simulink model "motor_model"  (R2022b)
settings: Solver=VariableStepAuto  StartTime=0.0  StopTime=5  FixedStep=Ts  RelTol=1e-3
undefined symbols (not defined in the file): DiscIntNeverNeededParam, param
settings Model: Creator=adelk  LastModifiedBy=adelk

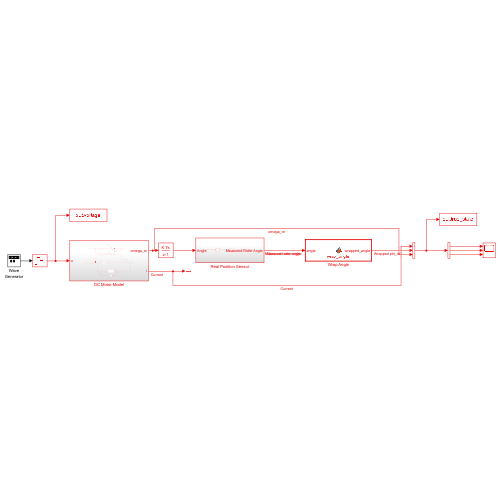
[thumbnail: Simulink's stored preview of the top-level diagram]
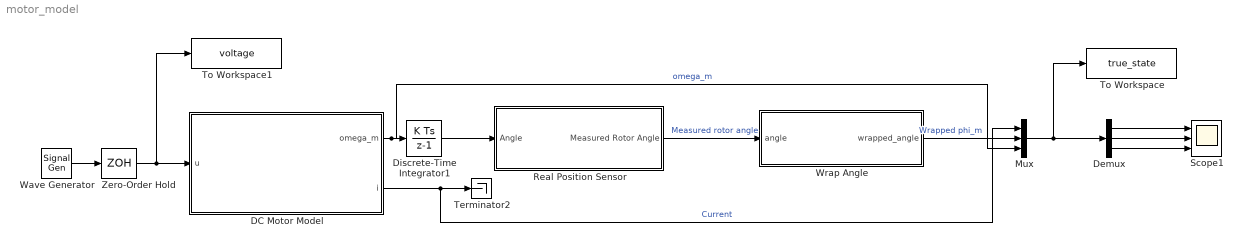
== system motor_model ==
  DC Motor Model : Subsystem
  Demux : Demux  Outputs=3
  Discrete-Time Integrator1 : DiscreteIntegrator  SampleTime=param.Ts  ICPrevOutput=DiscIntNeverNeededParam  ICPrevScaledInput=DiscIntNeverNeededParam
  Mux : Mux  Inputs=3
  Real Position Sensor : Subsystem
  Scope1 : Scope  NumInputPorts=3
  Terminator2 : Terminator
  To Workspace : ToWorkspace  VariableName=true_state  SampleTime=param.Ts
      settings: Save2DSignal=2-D array (concatenate along first dimension)
  To Workspace1 : ToWorkspace  VariableName=voltage  SampleTime=param.Ts
      settings: Save2DSignal=2-D array (concatenate along first dimension)
  Wave Generator : SignalGenerator  WaveForm=square  Amplitude=24  Frequency=50  Units=rad/sec
  Wrap Angle : MATLAB Function  TreatAsAtomicUnit=on
  Zero-Order Hold : ZeroOrderHold  SampleTime=param.Ts
  wires:
  DC Motor Model/1(omega_m) -> Mux/3, Discrete-Time Integrator1/1  "omega_m"
  DC Motor Model/2(i) -> Mux/1, Terminator2/1  "Current"
  Discrete-Time Integrator1/1 -> Real Position Sensor/1(Angle)
  Zero-Order Hold/1 -> To Workspace1/1, DC Motor Model/1(u)
  Real Position Sensor/1(Measured Rotor Angle) -> Wrap Angle/1(angle)  "Measured rotor angle"
  Mux/1 -> Demux/1, To Workspace/1
  Demux/1 -> Scope1/1
  Demux/2 -> Scope1/2
  Demux/3 -> Scope1/3
  Wrap Angle/1(wrapped_angle) -> Mux/2  "Wrapped phi_m"
  Wave Generator/1 -> Zero-Order Hold/1

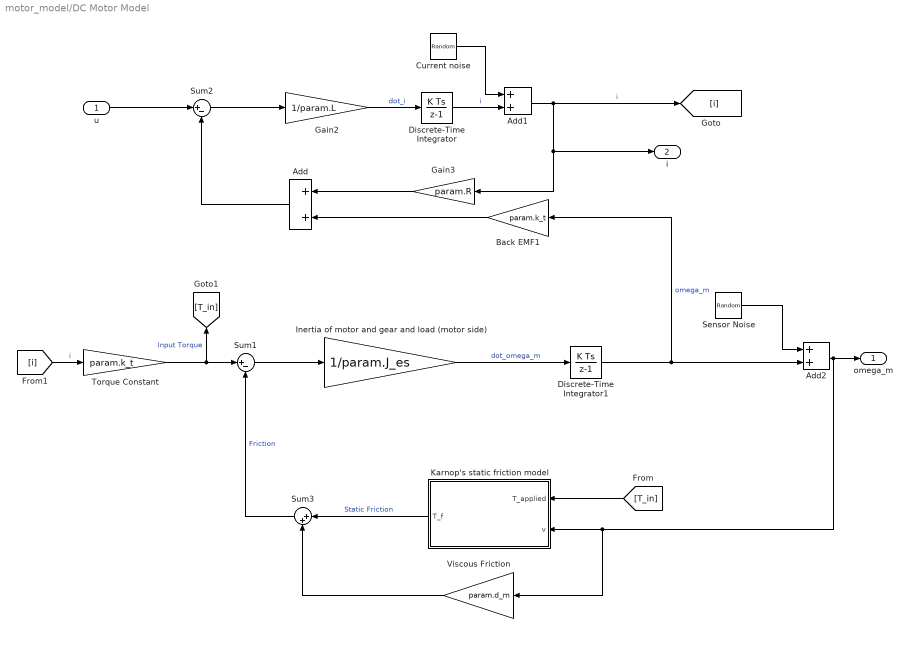
== system motor_model/DC Motor Model ==
  u : Inport
  Add : Sum
  Add1 : Sum
  Add2 : Sum
  Back EMF1 : Gain  Gain=param.k_t
  Current noise : RandomNumber  Variance=param.std_current_noise  SampleTime=param.Ts
  Discrete-Time Integrator : DiscreteIntegrator  SampleTime=param.Ts  ICPrevOutput=DiscIntNeverNeededParam  ICPrevScaledInput=DiscIntNeverNeededParam
  Discrete-Time Integrator1 : DiscreteIntegrator  SampleTime=param.Ts  ICPrevOutput=DiscIntNeverNeededParam  ICPrevScaledInput=DiscIntNeverNeededParam
  Gain2 : Gain  Gain=1/param.L
  Gain3 : Gain  Gain=param.R
  Inertia of motor and gear and load (motor side) : Gain  Gain=1/param.J_es
  Karnop's static friction model : Subsystem
  Sensor Noise : RandomNumber  Variance=param.std_encoder_noise  SampleTime=param.Ts
  Sum1 : Sum  Inputs=|+-
  Sum2 : Sum  Inputs=|+-
  Sum3 : Sum  Inputs=|++
  Torque Constant : Gain  Gain=param.k_t
  Viscous Friction : Gain  Gain=param.d_m
  omega_m : Outport
  i : Outport  Port=2
  wires:
  Add/1 -> Sum2/2
  Back EMF1/1 -> Add/2
  Gain3/1 -> Add/1
  Sum2/1 -> Gain2/1
  Add1/1 -> [i], Gain3/1, i/1  "i"
  Gain2/1 -> Discrete-Time Integrator/1  "dot_i"
  Inertia of motor and gear and load (motor side)/1 -> Discrete-Time Integrator1/1  "dot_omega_m"
  Discrete-Time Integrator1/1 -> Add2/2, Back EMF1/1  "omega_m"
  Torque Constant/1 -> [T_in], Sum1/1  "Input Torque"
  Viscous Friction/1 -> Sum3/2
  Sum1/1 -> Inertia of motor and gear and load (motor side)/1
  [i] -> Torque Constant/1  "i"
  Karnop's static friction model/1(T_f) -> Sum3/1  "Static Friction"
  Sum3/1 -> Sum1/2  "Friction"
  [T_in] -> Karnop's static friction model/1(T_applied)
  u/1 -> Sum2/1
  Discrete-Time Integrator/1 -> Add1/2  "i"
  Current noise/1 -> Add1/1
  Sensor Noise/1 -> Add2/1
  Add2/1 -> Viscous Friction/1, Karnop's static friction model/2(v), omega_m/1

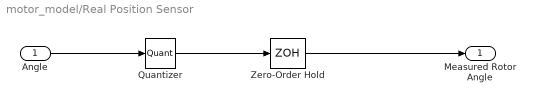
== system motor_model/Real Position Sensor ==
  Angle : Inport
  Quantizer : Quantizer  QuantizationInterval=param.quant_interval
  Zero-Order Hold : ZeroOrderHold  SampleTime=param.Ts
  Measured Rotor Angle : Outport
  wires:
  Zero-Order Hold/1 -> Measured Rotor Angle/1
  Quantizer/1 -> Zero-Order Hold/1
  Angle/1 -> Quantizer/1

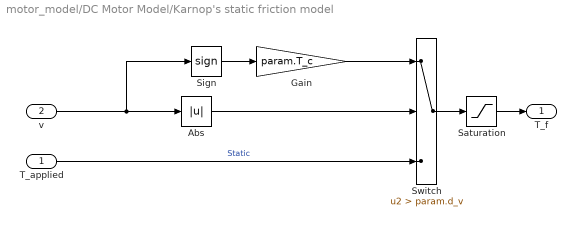
== system motor_model/DC Motor Model/Karnop's static friction model ==
  T_applied : Inport
  v : Inport  Port=2
  Abs : Abs  SaturateOnIntegerOverflow=off
  Gain : Gain  Gain=param.T_c
  Saturation : Saturate  UpperLimit=param.T_c  LowerLimit=-param.T_c
  Sign : Signum
  Switch : Switch  Criteria=u2 > Threshold  Threshold=param.d_v  ZeroCross=off  SaturateOnIntegerOverflow=off  InputSameDT=off
  T_f : Outport
  wires:
  Sign/1 -> Gain/1
  Abs/1 -> Switch/2
  T_applied/1 -> Switch/3  "Static"
  Switch/1 -> Saturation/1
  Saturation/1 -> T_f/1
  v/1 -> Abs/1, Sign/1
  Gain/1 -> Switch/1

== matlab function motor_model/Wrap Angle ==
  data: angle input; wrapped_angle output
function wrapped_angle = wrap_angle(angle)
wrapped_angle = mod(angle+pi,2*pi)- pi;
end
